simulink model "tutorial33_ukf"  (R2025a)
settings: Solver=VariableStepAuto  StartTime=0.0  StopTime=10.0  RelTol=1e-3
libraries: simulink x1
settings Model: Creator=xing2  LastModifiedBy=xing2

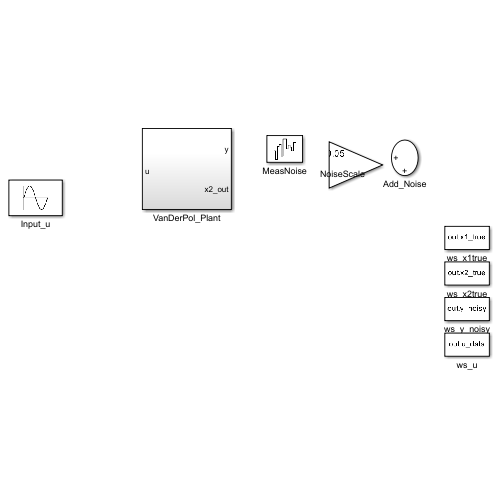
[thumbnail: Simulink's stored preview of the top-level diagram]
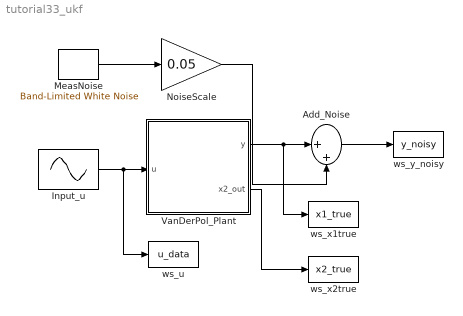
== system tutorial33_ukf ==
  Add_Noise : Sum  Inputs=|++
  Input_u : Sin  Amplitude=0.5  Frequency=0.8  SampleTime=0
  MeasNoise : simulink/Sources/Band-Limited White Noise  Cov=[0.1]  Ts=0.1  seed=[23341]
  NoiseScale : Gain  Gain=0.05
  VanDerPol_Plant : Subsystem
  ws_u : ToWorkspace  VariableName=u_data  SaveFormat=Timeseries  SampleTime=-1
  ws_x1true : ToWorkspace  VariableName=x1_true  SaveFormat=Timeseries  SampleTime=-1
  ws_x2true : ToWorkspace  VariableName=x2_true  SaveFormat=Timeseries  SampleTime=-1
  ws_y_noisy : ToWorkspace  VariableName=y_noisy  SaveFormat=Timeseries  SampleTime=-1
  wires:
  NoiseScale/1 -> Add_Noise/2
  MeasNoise/1 -> NoiseScale/1
  Input_u/1 -> VanDerPol_Plant/1(u), ws_u/1
  VanDerPol_Plant/2(x2_out) -> ws_x2true/1
  VanDerPol_Plant/1(y) -> ws_x1true/1, Add_Noise/1
  Add_Noise/1 -> ws_y_noisy/1

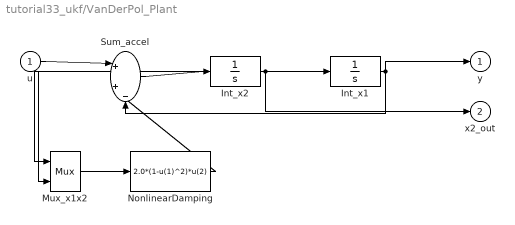
== system tutorial33_ukf/VanDerPol_Plant ==
  u : Inport
  Int_x1 : Integrator  InitialCondition=0.8
  Int_x2 : Integrator  InitialCondition=0.5
  Mux_x1x2 : Mux  Inputs=2
  NonlinearDamping : Fcn  Expr=2.0*(1-u(1)^2)*u(2)
  Sum_accel : Sum  Inputs=|++-
  y : Outport
  x2_out : Outport  Port=2
  wires:
  u/1 -> Sum_accel/1
  Sum_accel/1 -> Int_x2/1
  Int_x2/1 -> Int_x1/1, Mux_x1x2/2, x2_out/1
  Int_x1/1 -> Mux_x1x2/1, Sum_accel/3, y/1
  Mux_x1x2/1 -> NonlinearDamping/1
  NonlinearDamping/1 -> Sum_accel/2
